simulink model "PP"  (R2024b)
settings: Solver=ode3  StartTime=0.0  StopTime=10.0  FixedStep=0.1  RelTol=1e-3
settings Model: Creator=simon  LastModifiedBy=simon

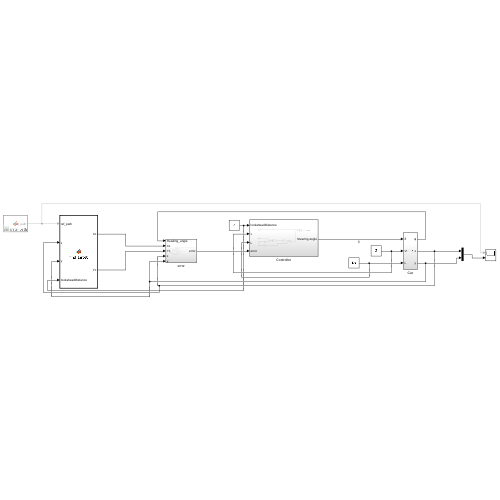
[thumbnail: Simulink's stored preview of the top-level diagram]
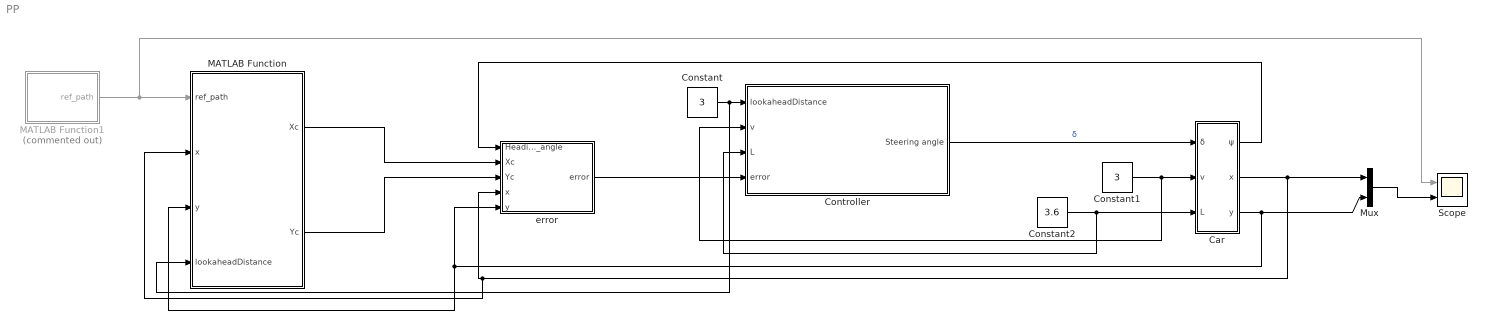
== system PP ==
  Car : Subsystem
  Constant : Constant  Value=3
  Constant1 : Constant  Value=3
  Constant2 : Constant  Value=3.6
  Controller : Subsystem
  MATLAB Function : MATLAB Function  TreatAsAtomicUnit=on
  MATLAB Function1 : MATLAB Function  Commented=on  TreatAsAtomicUnit=on
  Mux : Mux  Inputs=2
  Scope : Scope  NumInputPorts=2
  error : Subsystem
  wires:
  Controller/1(Steering angle) -> Car/1(δ)  "δ"
  Car/1(ψ) -> error/1(Heading_angle)
  error/1(error) -> Controller/4(error)
  Car/2(x) -> Mux/1, error/4(x), MATLAB Function/2(x)
  Car/3(y) -> error/5(y), MATLAB Function/3(y), Mux/2
  MATLAB Function/2(Yc) -> error/3(Yc)
  MATLAB Function/1(Xc) -> error/2(Xc)
  MATLAB Function1/1(ref_path) -> Scope/1, MATLAB Function/1(ref_path)
  Mux/1 -> Scope/2
  Constant/1 -> MATLAB Function/4(lookaheadDistance), Controller/1(lookaheadDistance)
  Constant1/1 -> Controller/2(v), Car/2(v)
  Constant2/1 -> Controller/3(L), Car/3(L)

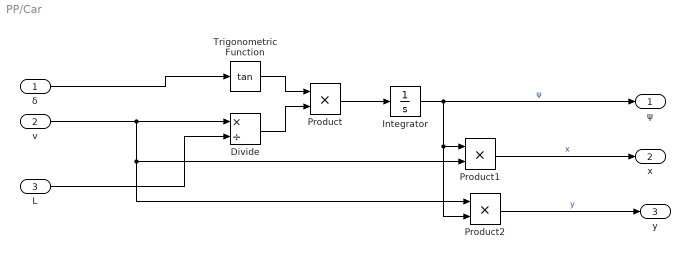
== system PP/Car ==
  δ : Inport
  v : Inport  Port=2
  L : Inport  Port=3
  Divide : Product  Inputs=*/
  Integrator : Integrator
  Product : Product
  Product1 : Product
  Product2 : Product
  Trigonometric Function : Trigonometry  Operator=tan
  ψ : Outport
  x : Outport  Port=2
  y : Outport  Port=3
  wires:
  δ/1 -> Trigonometric Function/1
  Divide/1 -> Product/2
  Product1/1 -> x/1  "x"
  Trigonometric Function/1 -> Product/1
  Product2/1 -> y/1  "y"
  L/1 -> Divide/2
  Product/1 -> Integrator/1
  Integrator/1 -> ψ/1, Product2/2, Product1/1  "ψ"
  v/1 -> Product2/1, Product1/2, Divide/1

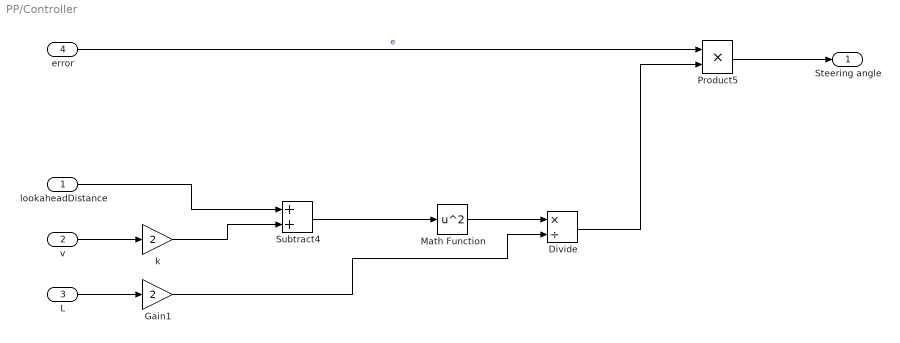
== system PP/Controller ==
  lookaheadDistance : Inport
  v : Inport  Port=2
  L : Inport  Port=3
  error : Inport  Port=4
  Divide : Product  Inputs=*/
  Gain1 : Gain  Gain=2
  Math Function : Math  Operator=square
  Product5 : Product
  Subtract4 : Sum
  k : Gain  Gain=2
  Steering angle : Outport  VectorParamsAs1DForOutWhenUnconnected=off
  wires:
  L/1 -> Gain1/1
  v/1 -> k/1
  Math Function/1 -> Divide/1
  k/1 -> Subtract4/2
  Divide/1 -> Product5/2
  Subtract4/1 -> Math Function/1
  Gain1/1 -> Divide/2
  lookaheadDistance/1 -> Subtract4/1
  Product5/1 -> Steering angle/1
  error/1 -> Product5/1  "e"

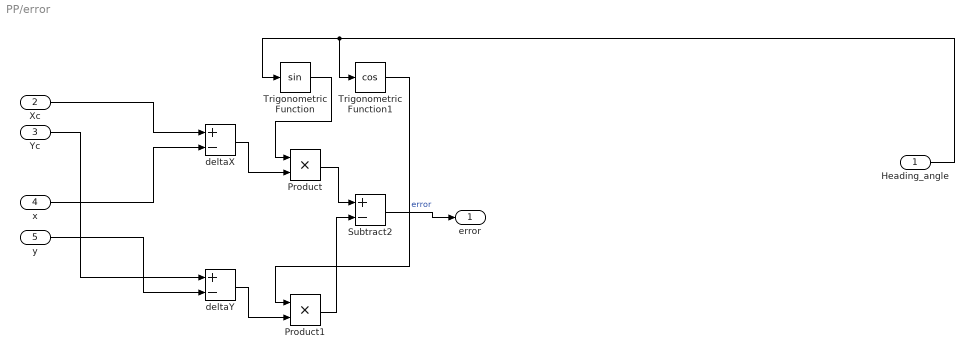
== system PP/error ==
  Heading_angle : Inport
  Xc : Inport  Port=2
  Yc : Inport  Port=3
  x : Inport  Port=4
  y : Inport  Port=5
  Product : Product
  Product1 : Product
  Subtract2 : Sum  Inputs=+-
  Trigonometric Function : Trigonometry
  Trigonometric Function1 : Trigonometry  Operator=cos
  deltaX : Sum  Inputs=+-
  deltaY : Sum  Inputs=+-
  error : Outport
  wires:
  deltaY/1 -> Product1/2
  Heading_angle/1 -> Trigonometric Function1/1, Trigonometric Function/1
  x/1 -> deltaX/2
  Xc/1 -> deltaX/1
  Trigonometric Function1/1 -> Product1/1
  Subtract2/1 -> error/1  "error"
  Product/1 -> Subtract2/1
  deltaX/1 -> Product/2
  Trigonometric Function/1 -> Product/1
  y/1 -> deltaY/2
  Product1/1 -> Subtract2/2
  Yc/1 -> deltaY/1

== matlab function PP/MATLAB Function1 ==
  data: ref_path output
function ref_path = generate_path()
    x = 0:0.1:10;        % start,step,stop
    A = 2.0;               % 振幅：2米
    omega = 0.5;         % 角频率：0.5 rad/m
    y = A * sin(omega * x);  % 正弦函数
    
    ref_path = [x', y'];  % 转换为 N×2 矩阵
end

== matlab function PP/MATLAB Function ==
  data: ref_path input; Xc output; x input; y input; lookaheadDistance input; Yc output
function [Xc, Yc] = find_target(ref_path, x, y, lookaheadDistance)
    % ref_path: 参考轨迹点，格式为 N×2 矩阵 [X1,Y1; X2,Y2; ...]
    % x, y: 车辆当前位置
    % lookaheadDistance: 预瞄距离 l_d
    
    N = size(ref_path, 1);% 返回矩阵的第一个维度(行)
    min_dist = Inf;
    Xc = 0;
    Yc = 0;
    
    for i = 1:N
        dx = ref_path(i, 1) - x;
        dy = ref_path(i, 2) - y;
        dist = sqrt(dx^2 + dy^2);
        
        % 找到距离最接近 lookaheadDistance 的点
        if abs(dist - lookaheadDistance) < min_dist
            min_dist = abs(dist - lookaheadDistance);
            Xc = ref_path(i, 1);
            Yc = ref_path(i, 2);
        end
    end
end
